simulink model "MIT_first_order"  (R2023a)
settings: Solver=FixedStepAuto  StartTime=start_time  StopTime=stop_time  FixedStep=sample_time  RelTol=1e-3
values from neighbouring files (symbols this model uses):
  a = 1    [example2.m]
  am = 2    [example2.m]
  b = 0.5    [example2.m]
  bm = 2    [example2.m]
  lambda = Lambda(i)    [example1.m]    (also in example2.m = 1)
  stop_time = 100.0    (= 100)    [Lyapunov_rule_order2.m]    (also in example1.m = 20; example2.m = 500)
libraries: simulink x1
settings Model: Creator=Mmoha  LastModifiedBy=Mmoha

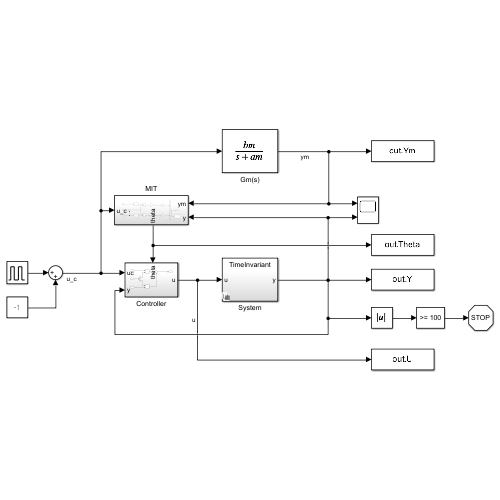
[thumbnail: Simulink's stored preview of the top-level diagram]
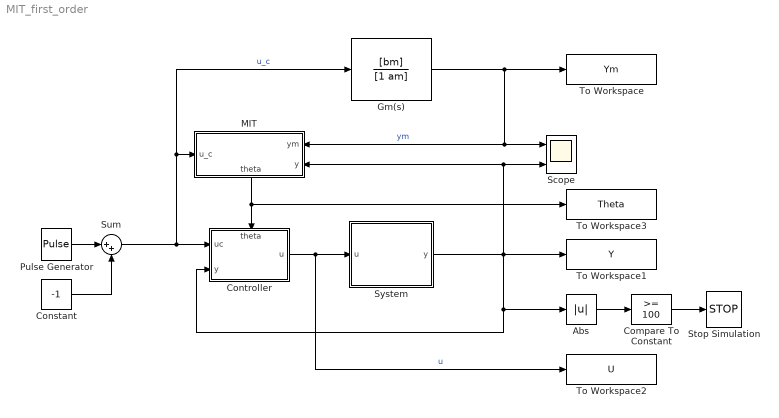
== system MIT_first_order ==
  Abs : Abs  SaturateOnIntegerOverflow=off
  Compare To Constant : simulink/Logic and Bit Operations/Compare To Constant  relop=>=  const=100  OutDataTypeStr=boolean
  Constant : Constant  Value=-1
  Controller : Subsystem
      settings: PortSchema="{\"entries\":[{\"content\":{\"sides\":[{\"content\":{\"connectorIds\":[\"In1\",\"In2\"]},\"type\":\"ConnectorPlacement.EquallySpacedRectSide\",\"uuid\":\"d022c748-101c-4660-a3ab-3ab175440250\"},{\"content\":{\"connectorIds\":[\"Out1\"],\"side\":\"RIGHT\"},\"type\":\"ConnectorPlacement.EquallySpacedRectSide\",\"uuid\":\"095f090d-91cf-42c9-9b75-572471a2012a\"},{\"content\":{\"connectorIds\":[\"In3\"],\"side\":\"TOP\"},\"type\":\"ConnectorPlacement.EquallySpacedRectSide\",\"uuid\":\"5fd4c211-bd76-4ce0-9b8f-def5304fcc21\"}]},\"type\":\"ConnectorPlacement.EquallySpacedConnector\",\"uuid\":\"4aef6e98-c23d-418c-9a84-b4a701bd8357\"}],\"packageUris\":[\"http://schema.mathworks.com/mf0/Connector/R2020b\"],\"version\":\"1.0\"}"
  Gm(s) : TransferFcn  Numerator=[bm]  Denominator=[1 am]
  MIT : Subsystem
      settings: PortSchema="{\"entries\":[{\"content\":{\"sides\":[{\"content\":{\"connectorIds\":[\"In1\",\"In2\"]},\"type\":\"ConnectorPlacement.EquallySpacedRectSide\",\"uuid\":\"b0e139f4-a3e5-4429-8b9f-fb5f46f8f8e3\"},{\"content\":{\"connectorIds\":[\"In3\"],\"side\":\"RIGHT\"},\"type\":\"ConnectorPlacement.EquallySpacedRectSide\",\"uuid\":\"e3848565-b04e-4aec-b58f-f857d7acf1b5\"},{\"content\":{\"side\":\"TOP\"},\"type\":\"ConnectorPlacement.EquallySpacedRectSide\",\"uuid\":\"208f314c-6f91-4f6a-965a-377babbc0509\"},{\"content\":{\"connectorIds\":[\"Out1\"],\"side\":\"BOTTOM\"},\"type\":\"ConnectorPlacement.EquallySpacedRectSide\",\"uuid\":\"5c536cd3-dfc6-4a5c-87a5-4f0046cabf11\"}]},\"type\":\"ConnectorPlacement.EquallySpacedConnector\",\"uuid\":\"c012dfe6-4353-43f0-ba00-c0e9dad8875b\"}],\"packageUris\":[\"http://schema.mathworks.com/mf0/Connector/R2020b\"],\"version\":\"1.0\"}"
  Pulse Generator : DiscretePulseGenerator  PulseType=Time based  Amplitude=2  Period=20  PulseWidth=50
  Scope : Scope  NumInputPorts=2
  Stop Simulation : Stop
  Sum : Sum  Inputs=|++
  System : Subsystem  Variant=on  VariantControlMode=label  VariantControl=Choice  LabelModeActiveChoice=Invariant
  To Workspace : ToWorkspace  VariableName=Ym  SaveFormat=Timeseries  SampleTime=-1
  To Workspace1 : ToWorkspace  VariableName=Y  SaveFormat=Timeseries  SampleTime=-1
  To Workspace2 : ToWorkspace  VariableName=U  SaveFormat=Timeseries  SampleTime=-1
  To Workspace3 : ToWorkspace  VariableName=Theta  SaveFormat=Timeseries  SampleTime=-1
  wires:
  Pulse Generator/1 -> Sum/1
  Constant/1 -> Sum/2
  Sum/1 -> MIT/3(u_c), Gm(s)/1, Controller/1(uc)  "u_c"
  Gm(s)/1 -> To Workspace/1, Scope/1, MIT/1(ym)  "ym"
  Controller/1(u) -> To Workspace2/1, System/1(u)  "u"
  MIT/1(theta) -> To Workspace3/1, Controller/3(theta)
  Compare To Constant/1 -> Stop Simulation/1
  System/1(y) -> Abs/1, Controller/2(y), Scope/2, MIT/2(y), To Workspace1/1
  Abs/1 -> Compare To Constant/1

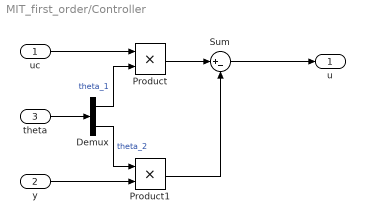
== system MIT_first_order/Controller ==
  uc : Inport
  y : Inport  Port=2
  theta : Inport  Port=3
  Demux : Demux  Outputs=2
  Product : Product
  Product1 : Product
  Sum : Sum  Inputs=|+-
  u : Outport
  wires:
  uc/1 -> Product/1
  y/1 -> Product1/2
  theta/1 -> Demux/1
  Demux/2 -> Product1/1  "theta_2"
  Product/1 -> Sum/1
  Product1/1 -> Sum/2
  Sum/1 -> u/1
  Demux/1 -> Product/2  "theta_1"

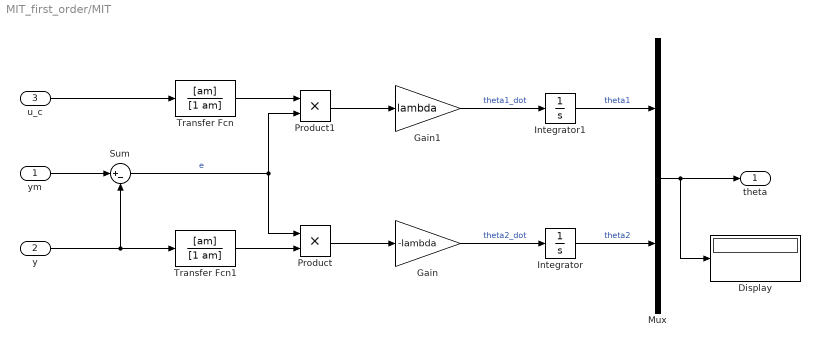
== system MIT_first_order/MIT ==
  ym : Inport
  y : Inport  Port=2
  u_c : Inport  Port=3
  Display : Display
  Gain : Gain  Gain=-lambda
  Gain1 : Gain  Gain=lambda
  Integrator : Integrator
  Integrator1 : Integrator
  Mux : Mux  Inputs=2
  Product : Product
  Product1 : Product
  Sum : Sum  Inputs=|+-
  Transfer Fcn : TransferFcn  Numerator=[am]  Denominator=[1 am]
  Transfer Fcn1 : TransferFcn  Numerator=[am]  Denominator=[1 am]
  theta : Outport
  wires:
  ym/1 -> Sum/1
  u_c/1 -> Transfer Fcn/1
  y/1 -> Sum/2, Transfer Fcn1/1
  Sum/1 -> Product1/2, Product/1  "e"
  Transfer Fcn1/1 -> Product/2
  Transfer Fcn/1 -> Product1/1
  Product/1 -> Gain/1
  Product1/1 -> Gain1/1
  Gain/1 -> Integrator/1  "theta2_dot"
  Gain1/1 -> Integrator1/1  "theta1_dot"
  Integrator/1 -> Mux/2  "theta2"
  Integrator1/1 -> Mux/1  "theta1"
  Mux/1 -> Display/1, theta/1

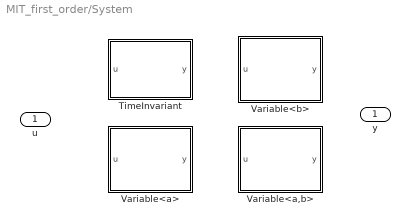
== system MIT_first_order/System ==
  u : Inport
  TimeInvariant : Subsystem  VariantControl=Invariant
  Variable<a,b> : Subsystem  VariantControl=Variable_a_b
  Variable<a> : Subsystem  VariantControl=Variable_a
  Variable<b> : Subsystem  VariantControl=Variable_b
  y : Outport

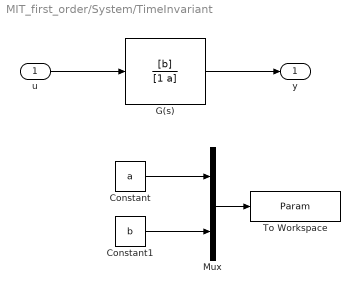
== system MIT_first_order/System/TimeInvariant ==
  u : Inport
  Constant : Constant  Value=a
  Constant1 : Constant  Value=b
  G(s) : TransferFcn  Numerator=[b]  Denominator=[1 a]
  Mux : Mux  Inputs=2
  To Workspace : ToWorkspace  VariableName=Param  SaveFormat=Timeseries  SampleTime=-1
  y : Outport
  wires:
  u/1 -> G(s)/1
  G(s)/1 -> y/1
  Mux/1 -> To Workspace/1
  Constant/1 -> Mux/1
  Constant1/1 -> Mux/2

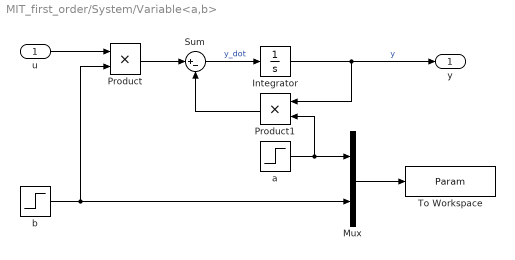
== system MIT_first_order/System/Variable<a,b> ==
  u : Inport
  Integrator : Integrator
  Mux : Mux  Inputs=2
  Product : Product
  Product1 : Product
  Sum : Sum  Inputs=|+-
  To Workspace : ToWorkspace  VariableName=Param  SaveFormat=Timeseries  SampleTime=-1
  a : Step  Time=stop_time/2  Before=1  After=2  SampleTime=0
  b : Step  Time=stop_time/2  Before=0.5  After=-0.5  SampleTime=0
  y : Outport
  wires:
  u/1 -> Product/1
  Product/1 -> Sum/1
  Sum/1 -> Integrator/1  "y_dot"
  Integrator/1 -> Product1/1, y/1  "y"
  Product1/1 -> Sum/2
  a/1 -> Product1/2, Mux/1
  b/1 -> Mux/2, Product/2
  Mux/1 -> To Workspace/1

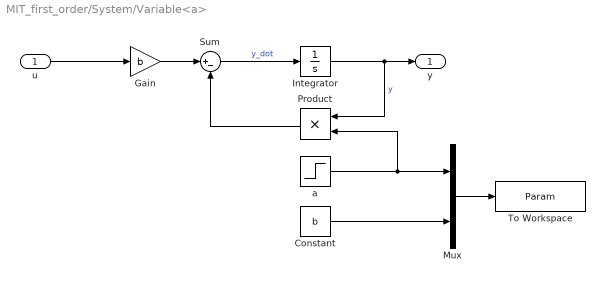
== system MIT_first_order/System/Variable<a> ==
  u : Inport
  Constant : Constant  Value=b
  Gain : Gain  Gain=b
  Integrator : Integrator
  Mux : Mux  Inputs=2
  Product : Product
  Sum : Sum  Inputs=|+-
  To Workspace : ToWorkspace  VariableName=Param  SaveFormat=Timeseries  SampleTime=-1
  a : Step  Time=stop_time/2  Before=1  After=2  SampleTime=0
  y : Outport
  wires:
  u/1 -> Gain/1
  Gain/1 -> Sum/1
  Sum/1 -> Integrator/1  "y_dot"
  Integrator/1 -> Product/1, y/1  "y"
  Product/1 -> Sum/2
  a/1 -> Product/2, Mux/1
  Mux/1 -> To Workspace/1
  Constant/1 -> Mux/2

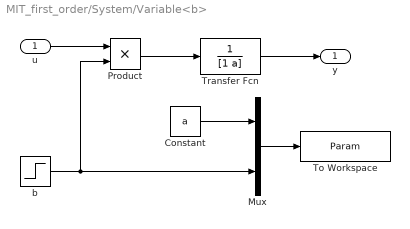
== system MIT_first_order/System/Variable<b> ==
  u : Inport
  Constant : Constant  Value=a
  Mux : Mux  Inputs=2
  Product : Product
  To Workspace : ToWorkspace  VariableName=Param  SaveFormat=Timeseries  SampleTime=-1
  Transfer Fcn : TransferFcn  Denominator=[1 a]
  b : Step  Time=stop_time/2  Before=0.5  After=-0.5  SampleTime=0
  y : Outport
  wires:
  u/1 -> Product/1
  Product/1 -> Transfer Fcn/1
  Transfer Fcn/1 -> y/1
  b/1 -> Mux/2, Product/2
  Mux/1 -> To Workspace/1
  Constant/1 -> Mux/1
